simulink model "sgMdl_CAN_CounterAndCRC"  (R2024b)
settings: Solver=FixedStepAuto  StartTime=0.0  StopTime=inf  RelTol=1e-3  EnableMultiTasking=on
undefined symbols (not defined in the file): CAN, Down, FD, Pull
libraries: CAN_message_utilities x14, canfdmsglib x10, speedgoatlib_IO602_4 x9, simulink x4
Description:
  | CAN - Counter and CRC Message Protection
settings Model: ModifiedByFormat=Speedgoat  SimulationMode=external  ExtModeEnableFloating=off  ExtModeTrigDuration=100000  Creator=Speedgoat  LastModifiedBy=Speedgoat
settings SolverCC: ConcurrentTasks=on  AlgebraicLoopSolver=TrustRegion  PositivePriorityOrder=on  AutoInsertRateTranBlk=on  InsertRTBMode=Never (minimum delay)
settings DataIOCC: SaveFormat=StructureWithTime
settings OptimizationCC: BlockReduction=off  OptimizeBlockIOStorage=off  BufferReuse=off  GlobalBufferReuse=off  ExpressionFolding=off  LocalBlockOutputs=off  OptimizeDataStoreBuffers=off  BusAssignmentInplaceUpdate=off
settings DebuggingCC: InheritedTsInSrcMsg=none  TasksWithSamePriorityMsg=none  ParameterPrecisionLossMsg=none  UnconnectedInputMsg=warning  UnconnectedOutputMsg=warning  UnconnectedLineMsg=warning
settings HardwareCC: ProdBitPerLong=64  ProdLongLongMode=on  ProdHWDeviceType=Intel->x86-64 (Linux 64)
settings ModelReferenceCC: EnableRefExpFcnMdlSchedulingChecks=on
settings SFSimCC: CustomCodeUndefinedFunction=UseInterfaceOnly
settings RTWCC: Description=Speedgoat Real-Time Target Machine  SystemTargetFile=speedgoat.tlc  TemplateMakefile=slrealtime_default_tmf  Toolchain=Simulink Real-Time Toolchain  BuildConfiguration=Faster Runs  TargetLang=C++  GPUComputeCapability=3.5  DLArmComputeVersion=19.05
settings SimulinkRealTimeTargetCC: SubcomponentCodeInterfacePackaging=Reusable function  InstructionSetFMA=off  LogToMDFFile=off  SLRTFileLogMaxRuns=10  UseGCCFastMath=on
settings ConfigComp: CovBoundaryAbsTol=1.0e-5

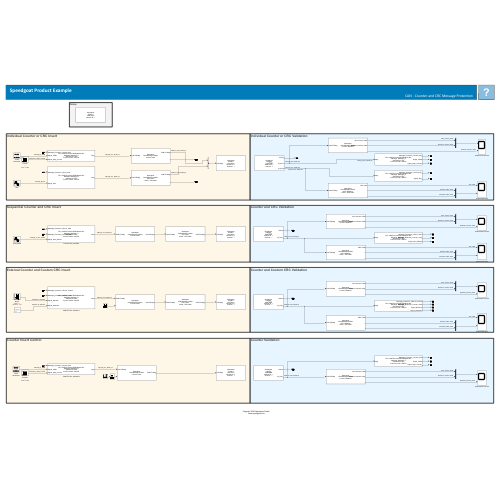
[thumbnail: Simulink's stored preview of the top-level diagram]
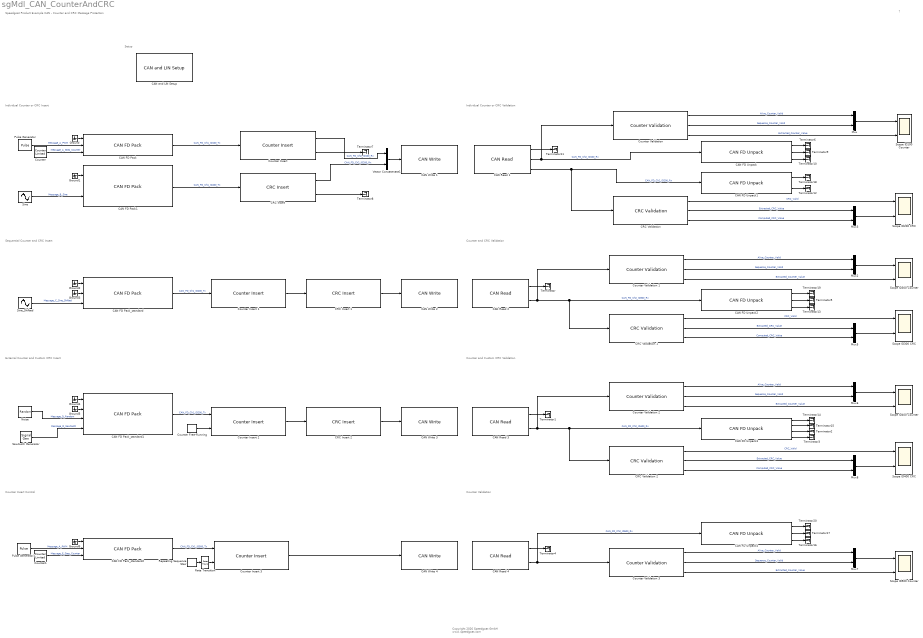
== system sgMdl_CAN_CounterAndCRC ==
  note: Individual Counter or CRC Insert
  note: Setup
  note: External Counter and Custom CRC Insert
  note: Counter Validation
  note: Individual Counter or CRC Validation
  note: Counter Insert Control
  note: Counter and CRC Validation
  note: Counter and Custom CRC Validation
  note: Sequential Counter and CRC Insert
  note: Speedgoat Product Example
      | CAN - Counter and CRC Message Protection
  note: ?
  note: Copyright 2026 Speedgoat GmbH
      |  www.speedgoat.com
  CAN FD Pack : canfdmsglib/CAN FD Pack  CANdbFile=CANFDCounterCRCDatabase.dbc  MsgList=Message_A  MsgName=Message_A  ProtocolMode=CAN FD  MsgIDType=Standard (11-bit identifier)  MsgIdentifier=100  CANIDInput=off  MsgLength=20  Remote=off  BRSSwitch=on  ApplyMinMax=off  SignalInfo={'Message_Protection_Counter_8bit','128','8','LE','unsigned','Standard','0','1','0','-Inf','Inf';'Signal_PWM','0','64','LE','double','Standard','0','1','0','-1.7e+308','1.7e+308';'Signal_Step_Counter','64','64','LE','double','Standard','0','1','0','-1.7e+308','1.7e+308'}
      settings: DataFormat=CANdb specified signals
  CAN FD Pack1 : canfdmsglib/CAN FD Pack  CANdbFile=CANFDCounterCRCDatabase.dbc  MsgList=Message_B  MsgName=Message_B  ProtocolMode=CAN FD  MsgIDType=Standard (11-bit identifier)  MsgIdentifier=200  CANIDInput=off  MsgLength=12  Remote=off  BRSSwitch=on  ApplyMinMax=off  SignalInfo={'Message_Protection_CRC8_0x2F','64','8','LE','unsigned','Standard','0','1','0','-Inf','Inf';'Signal_Sine','0','64','LE','double','Standard','0','1','0','-1.7e+308','1.7e+308'}
      settings: DataFormat=CANdb specified signals
  CAN FD Pack_standard : canfdmsglib/CAN FD Pack  CANdbFile=CANFDCounterCRCDatabase.dbc  MsgList=Message_C  MsgName=Message_C  ProtocolMode=CAN FD  MsgIDType=Standard (11-bit identifier)  MsgIdentifier=300  CANIDInput=off  MsgLength=12  Remote=off  BRSSwitch=on  ApplyMinMax=off  SignalInfo={'Message_Protection_CRC16_ARC','76','16','LE','unsigned','Standard','0','1','0','-Inf','Inf';'Message_Protection_Counter_12bit','64','12','LE','unsigned','Standard','0','1','0','-Inf','Inf';'Signal_Sine_Shifted','0','64','LE','double','Standard','0','1','0','-1.7e+308','1.7e+308'}
      settings: DataFormat=CANdb specified signals
  CAN FD Pack_standard1 : canfdmsglib/CAN FD Pack  CANdbFile=CANFDCounterCRCDatabase.dbc  MsgList=Message_D  MsgName=Message_D  ProtocolMode=CAN FD  MsgIDType=Standard (11-bit identifier)  MsgIdentifier=400  CANIDInput=off  MsgLength=7  Remote=off  BRSSwitch=on  ApplyMinMax=off  SignalInfo={'Message_Protection_CRC12_Custom','36','12','LE','unsigned','Standard','0','1','0','-Inf','Inf';'Message_Protection_Counter_16bit','12','16','LE','unsigned','Standard','0','1','0','-Inf','Inf';'Signal_Random','0','12','LE','unsigned','Standard','0','1','0','0','65535';'Signal_Sawtooth','28','6','LE','signed','Standard','0','1','0','-128','127'}
      settings: DataFormat=CANdb specified signals
  CAN FD Pack_standard2 : canfdmsglib/CAN FD Pack  CANdbFile=CANFDCounterCRCDatabase.dbc  MsgList=Message_E  MsgName=Message_E  ProtocolMode=CAN FD  MsgIDType=Standard (11-bit identifier)  MsgIdentifier=500  CANIDInput=off  MsgLength=20  Remote=off  BRSSwitch=on  ApplyMinMax=off  SignalInfo={'Message_Protection_Counter_8bit','128','8','LE','unsigned','Standard','0','1','0','-Inf','Inf';'Signal_PWM','0','64','LE','double','Standard','0','1','0','-1.7e+308','1.7e+308';'Signal_Step_Counter','64','64','LE','double','Standard','0','1','0','-1.7e+308','1.7e+308'}
      settings: DataFormat=CANdb specified signals
  CAN FD Unpack : canfdmsglib/CAN FD Unpack  CANdbFile=CANFDCounterCRCDatabase.dbc  MsgList=Message_A  MsgName=Message_A  ProtocolMode=CAN FD  MsgIDType=Standard (11-bit identifier)  MsgIdentifier=100  MsgLength=20  SignalInfo={'Message_Protection_Counter_8bit','128','8','LE','unsigned','Standard','0','1','0','-Inf','Inf';'Signal_PWM','0','64','LE','double','Standard','0','1','0','-1.7e+308','1.7e+308';'Signal_Step_Counter','64','64','LE','double','Standard','0','1','0','-1.7e+308','1.7e+308'}  IDPort=off  TimestampPort=off  ErrorPort=off  RemotePort=off  LengthPort=off  StatusPort=off  BRSPort=off  ESIPort=off  DLCPort=off  ApplyMinMax=off
      settings: DataFormat=CANdb specified signals
  CAN FD Unpack1 : canfdmsglib/CAN FD Unpack  CANdbFile=CANFDCounterCRCDatabase.dbc  MsgList=Message_B  MsgName=Message_B  ProtocolMode=CAN FD  MsgIDType=Standard (11-bit identifier)  MsgIdentifier=200  MsgLength=12  SignalInfo={'Message_Protection_CRC8_0x2F','64','8','LE','unsigned','Standard','0','1','0','-Inf','Inf';'Signal_Sine','0','64','LE','double','Standard','0','1','0','-1.7e+308','1.7e+308'}  IDPort=off  TimestampPort=off  ErrorPort=off  RemotePort=off  LengthPort=off  StatusPort=off  BRSPort=off  ESIPort=off  DLCPort=off  ApplyMinMax=off
      settings: DataFormat=CANdb specified signals
  CAN FD Unpack2 : canfdmsglib/CAN FD Unpack  CANdbFile=CANFDCounterCRCDatabase.dbc  MsgList=Message_C  MsgName=Message_C  ProtocolMode=CAN FD  MsgIDType=Standard (11-bit identifier)  MsgIdentifier=300  MsgLength=12  SignalInfo={'Message_Protection_CRC16_ARC','76','16','LE','unsigned','Standard','0','1','0','-Inf','Inf';'Message_Protection_Counter_12bit','64','12','LE','unsigned','Standard','0','1','0','-Inf','Inf';'Signal_Sine_Shifted','0','64','LE','double','Standard','0','1','0','-1.7e+308','1.7e+308'}  IDPort=off  TimestampPort=off  ErrorPort=off  RemotePort=off  LengthPort=off  StatusPort=off  BRSPort=off  ESIPort=off  DLCPort=off  ApplyMinMax=off
      settings: DataFormat=CANdb specified signals
  CAN FD Unpack3 : canfdmsglib/CAN FD Unpack  CANdbFile=CANFDCounterCRCDatabase.dbc  MsgList=Message_D  MsgName=Message_D  ProtocolMode=CAN FD  MsgIDType=Standard (11-bit identifier)  MsgIdentifier=400  MsgLength=7  SignalInfo={'Message_Protection_CRC12_Custom','36','12','LE','unsigned','Standard','0','1','0','-Inf','Inf';'Message_Protection_Counter_16bit','12','16','LE','unsigned','Standard','0','1','0','-Inf','Inf';'Signal_Random','0','12','LE','unsigned','Standard','0','1','0','0','65535';'Signal_Sawtooth','28','6','LE','signed','Standard','0','1','0','-128','127'}  IDPort=off  TimestampPort=off  ErrorPort=off  RemotePort=off  LengthPort=off  StatusPort=off  BRSPort=off  ESIPort=off  DLCPort=off  ApplyMinMax=off
      settings: DataFormat=CANdb specified signals
  CAN FD Unpack4 : canfdmsglib/CAN FD Unpack  CANdbFile=CANFDCounterCRCDatabase.dbc  MsgList=Message_E  MsgName=Message_E  ProtocolMode=CAN FD  MsgIDType=Standard (11-bit identifier)  MsgIdentifier=500  MsgLength=20  SignalInfo={'Message_Protection_Counter_8bit','128','8','LE','unsigned','Standard','0','1','0','-Inf','Inf';'Signal_PWM','0','64','LE','double','Standard','0','1','0','-1.7e+308','1.7e+308';'Signal_Step_Counter','64','64','LE','double','Standard','0','1','0','-1.7e+308','1.7e+308'}  IDPort=off  TimestampPort=off  ErrorPort=off  RemotePort=off  LengthPort=off  StatusPort=off  BRSPort=off  ESIPort=off  DLCPort=off  ApplyMinMax=off
      settings: DataFormat=CANdb specified signals
  CAN Read 1 : speedgoatlib_IO602_4/CAN Read   moduleType=IO603  id=1  channel=2  messageType=CAN-FD  useBusOut=on  HasMulRead=Specify by IDs  MsgIDlist=[100,200]  isEFF=off  LabelInHex=off  enableInput=off  initValues=[603 1 -1 1 2 0 1 2 0 2 100 200]  ts=-1
      settings: LibrarySourceBlock=speedgoatlib_IO602_IO691/CAN/CAN Read  SourceProductName=IO602-4
  CAN Read 2 : speedgoatlib_IO602_4/CAN Read   moduleType=IO603  id=1  channel=2  messageType=CAN-FD  useBusOut=on  HasMulRead=Specify by IDs  MsgIDlist=300  isEFF=off  LabelInHex=off  enableInput=off  initValues=[603 1 -1 1 2 0 1 2 0 1 300]  ts=-1
      settings: LibrarySourceBlock=speedgoatlib_IO602_IO691/CAN/CAN Read  SourceProductName=IO602-4
  CAN Read 3 : speedgoatlib_IO602_4/CAN Read   moduleType=IO603  id=1  channel=2  messageType=CAN-FD  useBusOut=on  HasMulRead=Specify by IDs  MsgIDlist=400  isEFF=off  LabelInHex=off  enableInput=off  initValues=[603 1 -1 1 2 0 1 2 0 1 400]  ts=-1
      settings: LibrarySourceBlock=speedgoatlib_IO602_IO691/CAN/CAN Read  SourceProductName=IO602-4
  CAN Read 4 : speedgoatlib_IO602_4/CAN Read   moduleType=IO603  id=1  channel=2  messageType=CAN-FD  useBusOut=on  HasMulRead=Specify by IDs  MsgIDlist=[500]  isEFF=off  LabelInHex=off  enableInput=off  initValues=[603 1 -1 1 2 0 1 2 0 1 500]  ts=-1
      settings: LibrarySourceBlock=speedgoatlib_IO602_IO691/CAN/CAN Read  SourceProductName=IO602-4
  CAN Write 1 : speedgoatlib_IO602_4/CAN Write   moduleType=IO603  id=1  channel=1  messageType=CAN-FD  useBusIn=on  numOfMsg=2  enableInput=off  enableStatusPort=off  ts=-1  initValues=[603 1 -1 0 2 0 2 0 1]
      settings: LibrarySourceBlock=speedgoatlib_IO602_IO691/CAN/CAN Write  SourceProductName=IO602-4
  CAN Write 2 : speedgoatlib_IO602_4/CAN Write   moduleType=IO603  id=1  channel=1  messageType=CAN-FD  useBusIn=on  numOfMsg=1  enableInput=off  enableStatusPort=off  ts=-1  initValues=[603 1 -1 0 2 0 1 0 1]
      settings: LibrarySourceBlock=speedgoatlib_IO602_IO691/CAN/CAN Write  SourceProductName=IO602-4
  CAN Write 3 : speedgoatlib_IO602_4/CAN Write   moduleType=IO603  id=1  channel=1  messageType=CAN-FD  useBusIn=on  numOfMsg=1  enableInput=off  enableStatusPort=off  ts=-1  initValues=[603 1 -1 0 2 0 1 0 1]
      settings: LibrarySourceBlock=speedgoatlib_IO602_IO691/CAN/CAN Write  SourceProductName=IO602-4
  CAN Write 4 : speedgoatlib_IO602_4/CAN Write   moduleType=IO603  id=1  channel=1  messageType=CAN-FD  useBusIn=on  numOfMsg=1  enableInput=off  enableStatusPort=off  ts=-1  initValues=[603 1 -1 0 2 0 1 0 1]
      settings: LibrarySourceBlock=speedgoatlib_IO602_IO691/CAN/CAN Write  SourceProductName=IO602-4
  "CAN and LIN Setup " : speedgoatlib_IO602_4/CAN and LIN Setup   moduleInitValues="[603    1    1   -1   -1]"  id=1  moduleType=IO603  pciSlot=-1  canChn1=CAN-FD  canChn2=CAN-FD  canChn3=Disabled  canChn4=Disabled  linChn1=Disabled  linChn2=Disabled  canInitStructArray=[]  canTermStructArray=[]  gpioChnx=Disabled  canChn1InitValues="[3   0   2   8  31   8  19   2   2   5   2   0]"  arbBdrChn1=1.0 MBaud  clockDividerChn1=Enable  arbManBdrChn1=[2,8,31,8]  fdBdrChn1=5.0 MBaud  fdManBdrChn1=[2,2,5,2]  termResistor1=off  canChn2InitValues="[3   0   2   8  31   8  19   2   2   5   2   0]"  arbBdrChn2=1.0 MBaud  clockDividerChn2=Enable  arbManBdrChn2=[2,8,31,8]  fdBdrChn2=5.0 MBaud  fdManBdrChn2=[2,2,5,2]  termResistor2=off  canChn3InitValues="[1   0   2   8  31   8  19   2   2   5   2   0]"  arbBdrChn3=1.0 MBaud  clockDividerChn3=Enable  arbManBdrChn3=[2,8,31,8]  fdBdrChn3=5.0 MBaud  fdManBdrChn3=[2,2,5,2]  termResistor3=off  canChn4InitValues="[1   0   2   8  31   8  19   2   2   5   2   0]"  arbBdrChn4=1.0 MBaud  clockDividerChn4=Enable  arbManBdrChn4=[2,8,31,8]  fdBdrChn4=5.0 MBaud  fdManBdrChn4=[2,2,5,2]  termResistor4=off  linChn1InitValues="[0  9600]"  linBtrChn1=9600  linChn2InitValues="[0  9600]"  linBtrChn2=9600  doInitTermStruct="[0  5  0  0  0]"  parDoChannels=[1 2]  parDoVoltage=5  parDoInitValues=0  parDoReset=1  parNumOfDoS=0  parDiChannels=[3 4]  parDiVoltage=5  parDiPull=Pull-Down
      settings: LibrarySourceBlock=speedgoatlib_IO602_IO691/CAN and LIN Setup  SourceProductName=IO602-4
  "CRC Insert " : CAN_message_utilities/CRC Insert   parEnableCrcPort=off  parCrcFromInput=off  parCrcOutput=on  parCrcType=CRC8 - 0x2F  parCrcBitLocation=64  parCustomCrcBitWidth=7  parCustomCrcFile=''  parCustomCrcFunction=''  parProtocol=CAN-FD  ts=-1  initValues=[0 2 47 255 255 0 0 64 1 7 2 -1]  lutParam=[0;47;94;113;188;147;226;205;87;120;9;38;235;196;181;154;174;129;240;223;18;61;76;99;249;214;167;136;69;106;27;52;115;92;45;2;207;224;145;190;36;11;122;85;152;183;198;233;221;242;131;172;97;78;63;16;138;165;212;251;54;25;104;71;230;201;184;151;90;117;4;43;177;158;239;192;13;34;83;124;72;103;22;57;244;219;170;133;31;48;65;110;163;140;253;210;149;186;203;228;41;6;119;88;194;237;156;179;126;81;32;15;59;20;101;74;135;168;217;246;108;67;50;29;208;255;142;161;227;204;189;146;95;112;1;46;180;155;234;197;8;39;86;121;77;98;19;60;241;222;175;128;26;53;68;107;166;137;248;215;144;191;206;225;44;3;114;93;199;232;153;182;123;84;37;10;62;17;96;79;130;173;220;243;105;70;55;24;213;250;139;164;5;42;91;116;185;150;231;200;82;125;12;35;238;193;176;159;171;132;245;218;23;56;73;102;252;211;162;141;64;111;30;49;118;89;40;7;202;229;148;187;33;14;127;80;157;178;195;236;216;247;134;169;100;75;58;21;143;160;209;254;51;28;109;66]
  CRC Insert 1 : CAN_message_utilities/CRC Insert   parEnableCrcPort=off  parCrcFromInput=off  parCrcOutput=off  parCrcType=CRC16 ARC  parCrcBitLocation=76  parCustomCrcBitWidth=7  parCustomCrcFile='test'  parCustomCrcFunction=''  parProtocol=CAN-FD  ts=-1  initValues=[0 5 32773 0 0 1 1 76 0 7 2 -1]  lutParam=[0;32773;32783;10;32795;30;20;32785;32819;54;60;32825;40;32813;32807;34;32867;102;108;32873;120;32893;32887;114;80;32853;32863;90;32843;78;68;32833;32963;198;204;32969;216;32989;32983;210;240;33013;33023;250;33003;238;228;32993;160;32933;32943;170;32955;190;180;32945;32915;150;156;32921;136;32909;32903;130;33155;390;396;33161;408;33181;33175;402;432;33205;33215;442;33195;430;420;33185;480;33253;33263;490;33275;510;500;33265;33235;470;476;33241;456;33229;33223;450;320;33093;33103;330;33115;350;340;33105;33139;374;380;33145;360;33133;33127;354;33059;294;300;33065;312;33085;33079;306;272;33045;33055;282;33035;270;260;33025;33539;774;780;33545;792;33565;33559;786;816;33589;33599;826;33579;814;804;33569;864;33637;33647;874;33659;894;884;33649;33619;854;860;33625;840;33613;33607;834;960;33733;33743;970;33755;990;980;33745;33779;1014;1020;33785;1000;33773;33767;994;33699;934;940;33705;952;33725;33719;946;912;33685;33695;922;33675;910;900;33665;640;33413;33423;650;33435;670;660;33425;33459;694;700;33465;680;33453;33447;674;33507;742;748;33513;760;33533;33527;754;720;33493;33503;730;33483;718;708;33473;33347;582;588;33353;600;33373;33367;594;624;33397;33407;634;33387;622;612;33377;544;33317;33327;554;33339;574;564;33329;33299;534;540;33305;520;33293;33287;514]
  CRC Insert 2 : CAN_message_utilities/CRC Insert   parEnableCrcPort=off  parCrcFromInput=on  parCrcOutput=off  parCrcType=Custom  parCrcBitLocation=36  parCustomCrcBitWidth=12  parCustomCrcFile='custom_crc.cpp'  parCustomCrcFunction='ComputeCustomCrc'  parProtocol=CAN-FD  ts=-1  initValues=[0 8 0 0 0 0 0 36 0 12 2 -1]  lutParam=[0;29;58;39;116;105;78;83;232;245;210;207;156;129;166;187;205;208;247;234;185;164;131;158;37;56;31;2;81;76;107;118;135;154;189;160;243;238;201;212;111;114;85;72;27;6;33;60;74;87;112;109;62;35;4;25;162;191;152;133;214;203;236;241;19;14;41;52;103;122;93;64;251;230;193;220;143;146;181;168;222;195;228;249;170;183;144;141;54;43;12;17;66;95;120;101;148;137;174;179;224;253;218;199;124;97;70;91;8;21;50;47;89;68;99;126;45;48;23;10;177;172;139;150;197;216;255;226;38;59;28;1;82;79;104;117;206;211;244;233;186;167;128;157;235;246;209;204;159;130;165;184;3;30;57;36;119;106;77;80;161;188;155;134;213;200;239;242;73;84;115;110;61;32;7;26;108;113;86;75;24;5;34;63;132;153;190;163;240;237;202;215;53;40;15;18;65;92;123;102;221;192;231;250;169;180;147;142;248;229;194;223;140;145;182;171;16;13;42;55;100;121;94;67;178;175;136;149;198;219;252;225;90;71;96;125;46;51;20;9;127;98;69;88;11;22;49;44;151;138;173;176;227;254;217;196]
  "CRC Validation " : CAN_message_utilities/CRC Validation   parEnableCrcPort=off  parCrcFromInput=off  parComputedCrcOutput=on  parExtractedCrcOutput=on  parCrcValidOutput=on  parCrcType=CRC8 - 0x2F  parCrcBitLocation=64  parCustomCrcBitWidth=8  parCustomCrcFile=''  parCustomCrcFunction=''  parProtocol=CAN-FD  ts=-1  initValues=[0 2 47 255 255 0 0 64 1 1 1 8 2 -1]  lutParam=[0;47;94;113;188;147;226;205;87;120;9;38;235;196;181;154;174;129;240;223;18;61;76;99;249;214;167;136;69;106;27;52;115;92;45;2;207;224;145;190;36;11;122;85;152;183;198;233;221;242;131;172;97;78;63;16;138;165;212;251;54;25;104;71;230;201;184;151;90;117;4;43;177;158;239;192;13;34;83;124;72;103;22;57;244;219;170;133;31;48;65;110;163;140;253;210;149;186;203;228;41;6;119;88;194;237;156;179;126;81;32;15;59;20;101;74;135;168;217;246;108;67;50;29;208;255;142;161;227;204;189;146;95;112;1;46;180;155;234;197;8;39;86;121;77;98;19;60;241;222;175;128;26;53;68;107;166;137;248;215;144;191;206;225;44;3;114;93;199;232;153;182;123;84;37;10;62;17;96;79;130;173;220;243;105;70;55;24;213;250;139;164;5;42;91;116;185;150;231;200;82;125;12;35;238;193;176;159;171;132;245;218;23;56;73;102;252;211;162;141;64;111;30;49;118;89;40;7;202;229;148;187;33;14;127;80;157;178;195;236;216;247;134;169;100;75;58;21;143;160;209;254;51;28;109;66]
  CRC Validation 1 : CAN_message_utilities/CRC Validation   parEnableCrcPort=off  parCrcFromInput=off  parComputedCrcOutput=on  parExtractedCrcOutput=on  parCrcValidOutput=on  parCrcType=CRC16 ARC  parCrcBitLocation=76  parCustomCrcBitWidth=8  parCustomCrcFile=''  parCustomCrcFunction=''  parProtocol=CAN-FD  ts=-1  initValues=[0 5 32773 0 0 1 1 76 1 1 1 8 2 -1]  lutParam=[0;32773;32783;10;32795;30;20;32785;32819;54;60;32825;40;32813;32807;34;32867;102;108;32873;120;32893;32887;114;80;32853;32863;90;32843;78;68;32833;32963;198;204;32969;216;32989;32983;210;240;33013;33023;250;33003;238;228;32993;160;32933;32943;170;32955;190;180;32945;32915;150;156;32921;136;32909;32903;130;33155;390;396;33161;408;33181;33175;402;432;33205;33215;442;33195;430;420;33185;480;33253;33263;490;33275;510;500;33265;33235;470;476;33241;456;33229;33223;450;320;33093;33103;330;33115;350;340;33105;33139;374;380;33145;360;33133;33127;354;33059;294;300;33065;312;33085;33079;306;272;33045;33055;282;33035;270;260;33025;33539;774;780;33545;792;33565;33559;786;816;33589;33599;826;33579;814;804;33569;864;33637;33647;874;33659;894;884;33649;33619;854;860;33625;840;33613;33607;834;960;33733;33743;970;33755;990;980;33745;33779;1014;1020;33785;1000;33773;33767;994;33699;934;940;33705;952;33725;33719;946;912;33685;33695;922;33675;910;900;33665;640;33413;33423;650;33435;670;660;33425;33459;694;700;33465;680;33453;33447;674;33507;742;748;33513;760;33533;33527;754;720;33493;33503;730;33483;718;708;33473;33347;582;588;33353;600;33373;33367;594;624;33397;33407;634;33387;622;612;33377;544;33317;33327;554;33339;574;564;33329;33299;534;540;33305;520;33293;33287;514]
  CRC Validation 2 : CAN_message_utilities/CRC Validation   parEnableCrcPort=off  parCrcFromInput=off  parComputedCrcOutput=on  parExtractedCrcOutput=on  parCrcValidOutput=on  parCrcType=Custom  parCrcBitLocation=36  parCustomCrcBitWidth=12  parCustomCrcFile='custom_crc.cpp'  parCustomCrcFunction='ComputeCustomCrc'  parProtocol=CAN-FD  ts=-1  initValues=[0 8 0 0 0 0 0 36 1 1 1 12 2 -1]  lutParam=[0;47;94;113;188;147;226;205;87;120;9;38;235;196;181;154;174;129;240;223;18;61;76;99;249;214;167;136;69;106;27;52;115;92;45;2;207;224;145;190;36;11;122;85;152;183;198;233;221;242;131;172;97;78;63;16;138;165;212;251;54;25;104;71;230;201;184;151;90;117;4;43;177;158;239;192;13;34;83;124;72;103;22;57;244;219;170;133;31;48;65;110;163;140;253;210;149;186;203;228;41;6;119;88;194;237;156;179;126;81;32;15;59;20;101;74;135;168;217;246;108;67;50;29;208;255;142;161;227;204;189;146;95;112;1;46;180;155;234;197;8;39;86;121;77;98;19;60;241;222;175;128;26;53;68;107;166;137;248;215;144;191;206;225;44;3;114;93;199;232;153;182;123;84;37;10;62;17;96;79;130;173;220;243;105;70;55;24;213;250;139;164;5;42;91;116;185;150;231;200;82;125;12;35;238;193;176;159;171;132;245;218;23;56;73;102;252;211;162;141;64;111;30;49;118;89;40;7;202;229;148;187;33;14;127;80;157;178;195;236;216;247;134;169;100;75;58;21;143;160;209;254;51;28;109;66]
  Counter : simulink/Sources/Counter Limited  uplimit=64  tsamp=10e-3
      settings: AttributesFormatString=|
      | ---
      | Limit: %<uplimit> bits
  Counter Free-Running : simulink/Sources/Counter Free-Running  NumBits=16  tsamp=10e-3
  "Counter Insert " : CAN_message_utilities/Counter Insert   parEnablePort=off  parCounterControlPort=off  parCounterFromInput=off  parCounterOutport=on  parCounterStart=1  parCounterStop=15  parCounterStep=1  parCounterBitLocation=128  parCounterLength=8  parProtocol=CAN-FD  ts=-1  initValues=[0 0 0 1 15 1 128 8 1 2 -1]
  Counter Insert 1 : CAN_message_utilities/Counter Insert   parEnablePort=off  parCounterControlPort=off  parCounterFromInput=off  parCounterOutport=off  parCounterStart=1  parCounterStop=4000  parCounterStep=3  parCounterBitLocation=64  parCounterLength=12  parProtocol=CAN-FD  ts=-1  initValues=[0 0 0 1 4000 3 64 12 0 2 -1]
  Counter Insert 2 : CAN_message_utilities/Counter Insert   parEnablePort=off  parCounterControlPort=off  parCounterFromInput=on  parCounterOutport=off  parCounterStart=1  parCounterStop=15  parCounterStep=1  parCounterBitLocation=12  parCounterLength=16  parProtocol=CAN-FD  ts=-1  initValues=[0 0 1 1 15 1 12 16 0 2 -1]
  Counter Insert 3 : CAN_message_utilities/Counter Insert   parEnablePort=off  parCounterControlPort=on  parCounterFromInput=off  parCounterOutport=off  parCounterStart=1  parCounterStop=15  parCounterStep=1  parCounterBitLocation=128  parCounterLength=8  parProtocol=CAN-FD  ts=-1  initValues=[0 1 0 1 15 1 128 8 0 2 -1]
  "Counter Validation " : CAN_message_utilities/Counter Validation   parExtractedCounterOutput=on  parAliveCounterValidOutput=on  parSequenceCounterValidOutput=on  parMissedFramesOutput=off  parCounterStartValue=1  parCounterStopValue=15  parCounterStepValue=1  parCounterBitLocation=128  parCounterBitWidth=8  parProtocol=CAN-FD  ts=-1  initValues=[1 15 1 128 8 1 1 1 0 2 -1]  lutParam=[0;29;58;39;116;105;78;83;232;245;210;207;156;129;166;187;205;208;247;234;185;164;131;158;37;56;31;2;81;76;107;118;135;154;189;160;243;238;201;212;111;114;85;72;27;6;33;60;74;87;112;109;62;35;4;25;162;191;152;133;214;203;236;241;19;14;41;52;103;122;93;64;251;230;193;220;143;146;181;168;222;195;228;249;170;183;144;141;54;43;12;17;66;95;120;101;148;137;174;179;224;253;218;199;124;97;70;91;8;21;50;47;89;68;99;126;45;48;23;10;177;172;139;150;197;216;255;226;38;59;28;1;82;79;104;117;206;211;244;233;186;167;128;157;235;246;209;204;159;130;165;184;3;30;57;36;119;106;77;80;161;188;155;134;213;200;239;242;73;84;115;110;61;32;7;26;108;113;86;75;24;5;34;63;132;153;190;163;240;237;202;215;53;40;15;18;65;92;123;102;221;192;231;250;169;180;147;142;248;229;194;223;140;145;182;171;16;13;42;55;100;121;94;67;178;175;136;149;198;219;252;225;90;71;96;125;46;51;20;9;127;98;69;88;11;22;49;44;151;138;173;176;227;254;217;196]
  Counter Validation 1 : CAN_message_utilities/Counter Validation   parExtractedCounterOutput=on  parAliveCounterValidOutput=on  parSequenceCounterValidOutput=on  parMissedFramesOutput=off  parCounterStartValue=1  parCounterStopValue=4000  parCounterStepValue=3  parCounterBitLocation=64  parCounterBitWidth=12  parProtocol=CAN-FD  ts=-1  initValues=[1 4000 3 64 12 1 1 1 0 2 -1]  lutParam=[0;29;58;39;116;105;78;83;232;245;210;207;156;129;166;187;205;208;247;234;185;164;131;158;37;56;31;2;81;76;107;118;135;154;189;160;243;238;201;212;111;114;85;72;27;6;33;60;74;87;112;109;62;35;4;25;162;191;152;133;214;203;236;241;19;14;41;52;103;122;93;64;251;230;193;220;143;146;181;168;222;195;228;249;170;183;144;141;54;43;12;17;66;95;120;101;148;137;174;179;224;253;218;199;124;97;70;91;8;21;50;47;89;68;99;126;45;48;23;10;177;172;139;150;197;216;255;226;38;59;28;1;82;79;104;117;206;211;244;233;186;167;128;157;235;246;209;204;159;130;165;184;3;30;57;36;119;106;77;80;161;188;155;134;213;200;239;242;73;84;115;110;61;32;7;26;108;113;86;75;24;5;34;63;132;153;190;163;240;237;202;215;53;40;15;18;65;92;123;102;221;192;231;250;169;180;147;142;248;229;194;223;140;145;182;171;16;13;42;55;100;121;94;67;178;175;136;149;198;219;252;225;90;71;96;125;46;51;20;9;127;98;69;88;11;22;49;44;151;138;173;176;227;254;217;196]
  Counter Validation 2 : CAN_message_utilities/Counter Validation   parExtractedCounterOutput=on  parAliveCounterValidOutput=on  parSequenceCounterValidOutput=on  parMissedFramesOutput=off  parCounterStartValue=0  parCounterStopValue=65535  parCounterStepValue=1  parCounterBitLocation=12  parCounterBitWidth=16  parProtocol=CAN-FD  ts=-1  initValues=[0 65535 1 12 16 1 1 1 0 2 -1]  lutParam=[0;29;58;39;116;105;78;83;232;245;210;207;156;129;166;187;205;208;247;234;185;164;131;158;37;56;31;2;81;76;107;118;135;154;189;160;243;238;201;212;111;114;85;72;27;6;33;60;74;87;112;109;62;35;4;25;162;191;152;133;214;203;236;241;19;14;41;52;103;122;93;64;251;230;193;220;143;146;181;168;222;195;228;249;170;183;144;141;54;43;12;17;66;95;120;101;148;137;174;179;224;253;218;199;124;97;70;91;8;21;50;47;89;68;99;126;45;48;23;10;177;172;139;150;197;216;255;226;38;59;28;1;82;79;104;117;206;211;244;233;186;167;128;157;235;246;209;204;159;130;165;184;3;30;57;36;119;106;77;80;161;188;155;134;213;200;239;242;73;84;115;110;61;32;7;26;108;113;86;75;24;5;34;63;132;153;190;163;240;237;202;215;53;40;15;18;65;92;123;102;221;192;231;250;169;180;147;142;248;229;194;223;140;145;182;171;16;13;42;55;100;121;94;67;178;175;136;149;198;219;252;225;90;71;96;125;46;51;20;9;127;98;69;88;11;22;49;44;151;138;173;176;227;254;217;196]
  Counter Validation 3 : CAN_message_utilities/Counter Validation   parExtractedCounterOutput=on  parAliveCounterValidOutput=on  parSequenceCounterValidOutput=on  parMissedFramesOutput=off  parCounterStartValue=1  parCounterStopValue=15  parCounterStepValue=1  parCounterBitLocation=128  parCounterBitWidth=8  parProtocol=CAN-FD  ts=-1  initValues=[1 15 1 128 8 1 1 1 0 2 -1]  lutParam=[0;29;58;39;116;105;78;83;232;245;210;207;156;129;166;187;205;208;247;234;185;164;131;158;37;56;31;2;81;76;107;118;135;154;189;160;243;238;201;212;111;114;85;72;27;6;33;60;74;87;112;109;62;35;4;25;162;191;152;133;214;203;236;241;19;14;41;52;103;122;93;64;251;230;193;220;143;146;181;168;222;195;228;249;170;183;144;141;54;43;12;17;66;95;120;101;148;137;174;179;224;253;218;199;124;97;70;91;8;21;50;47;89;68;99;126;45;48;23;10;177;172;139;150;197;216;255;226;38;59;28;1;82;79;104;117;206;211;244;233;186;167;128;157;235;246;209;204;159;130;165;184;3;30;57;36;119;106;77;80;161;188;155;134;213;200;239;242;73;84;115;110;61;32;7;26;108;113;86;75;24;5;34;63;132;153;190;163;240;237;202;215;53;40;15;18;65;92;123;102;221;192;231;250;169;180;147;142;248;229;194;223;140;145;182;171;16;13;42;55;100;121;94;67;178;175;136;149;198;219;252;225;90;71;96;125;46;51;20;9;127;98;69;88;11;22;49;44;151;138;173;176;227;254;217;196]
  Counter1 : simulink/Sources/Counter Limited  uplimit=64  tsamp=10e-3
      settings: AttributesFormatString=|
      | ---
      | Limit: %<uplimit> bits
  Ground{,1..6} (7 alike) : Ground
  Mux{,2..3,5..8} (7 alike) : Mux  Inputs=2
  Noise : RandomNumber  Variance=100  SampleTime=10e-3
      settings: AttributesFormatString=|
      | Mean: %<Mean>
      | Variance: %<Variance>
  Pulse Generator : DiscretePulseGenerator  Period=50  PulseWidth=20  SampleTime=10e-3
  Pulse Generator1 : DiscretePulseGenerator  Period=50  PulseWidth=20  SampleTime=10e-3
  Rate Transition : RateTransition
  Repeating Sequence Stair : simulink/Sources/Repeating Sequence Stair  OutValues=[1 0 5 0xFFFF].'  tsamp=1  OutMin=[]  OutMax=[]  OutDataTypeStr=uint32  OutputDataTypeScalingMode=uint32  OutDataType=fixdt(0,8)  ConRadixGroup=Best Precision: Vector-wise  OutScaling=2^-12
  Sawtooth Generator : SignalGenerator  WaveForm=sawtooth  Amplitude=63  Frequency=5
  Scope ID100 Counter : Scope  NumInputPorts=2
  Scope ID200 CRC : Scope  NumInputPorts=2
  Scope ID300 CRC : Scope  NumInputPorts=2
  Scope ID300 Counter : Scope  NumInputPorts=2
  Scope ID400 CRC : Scope  NumInputPorts=2
  Scope ID400 Counter : Scope  NumInputPorts=2
  Scope ID500 Counter : Scope  NumInputPorts=2
  Sine : Sin  Amplitude=255  Frequency=2*pi  SampleTime=10e-3
  Sine_Shifted : Sin  Amplitude=255  Bias=pi  Frequency=2*pi  SampleTime=10e-3
  Terminator{,1..20} (21 alike) : Terminator
  Vector Concatenate1 : Concatenate
  wires:
  "Counter Validation "/3 -> Scope ID100 Counter/2  "Extracted_Counter_Value"
  CRC Validation 1/2 -> Mux5/1  "Extracted_CRC_Value"
  "CRC Validation "/1 -> Scope ID200 CRC/1  "CRC_Valid"
  CAN FD Unpack2/3 -> Terminator13/1
  CAN Read 3/1 -> Terminator1/1
  CAN Read 2/2 -> CRC Validation 1/1, CAN FD Unpack2/1, Counter Validation 1/1  "CAN_FD_Ch2_ID300_Rx"
  CAN FD Unpack/2 -> Terminator9/1
  CAN Read 1/2 -> "Counter Validation "/1, CAN FD Unpack/1  "CAN_FD_Ch2_ID100_Rx"
  CAN Read 1/1 -> Terminator11/1
  CAN FD Pack_standard1/1 -> Counter Insert 2/1  "CAN_FD_Ch1_ID200_Tx"
  CAN FD Unpack/1 -> Terminator6/1
  Pulse Generator/1 -> CAN FD Pack/2  "Message_A_PWM"
  CAN FD Pack1/1 -> "CRC Insert "/1  "CAN_FD_Ch1_ID400_Tx"
  CRC Validation 1/1 -> Scope ID300 CRC/1  "CRC_Valid"
  Counter/1 -> CAN FD Pack/3  "Message_A_Step_Counter"
  "Counter Insert "/2 -> Terminator7/1
  "CRC Validation "/2 -> Mux3/1  "Extracted_CRC_Value"
  Counter Validation 2/2 -> Mux6/2  "Sequence_Counter_Valid"
  Counter Validation 1/1 -> Mux2/1  "Alive_Counter_Valid"
  Noise/1 -> CAN FD Pack_standard1/3  "Message_D_Random"
  Mux6/1 -> Scope ID400 Counter/1
  CAN Read 2/1 -> Terminator/1
  Ground5/1 -> CAN FD Pack_standard1/2
  Ground2/1 -> CAN FD Pack_standard/1
  Counter Validation 2/1 -> Mux6/1  "Alive_Counter_Valid"
  Sine_Shifted/1 -> CAN FD Pack_standard/3  "Message_C_Sine_Shifted"
  CRC Validation 2/3 -> Mux8/2  "Computed_CRC_Value"
  CAN FD Unpack3/3 -> Terminator2/1
  Mux/1 -> Scope ID100 Counter/1
  Mux2/1 -> Scope ID300 Counter/1
  CAN FD Unpack3/1 -> Terminator14/1
  Ground1/1 -> CAN FD Pack1/1
  "CRC Validation "/3 -> Mux3/2  "Computed_CRC_Value"
  Sine/1 -> CAN FD Pack1/2  "Message_B_Sine"
  CAN FD Pack_standard/1 -> Counter Insert 1/1  "CAN_FD_Ch1_ID200_Tx"
  Ground3/1 -> CAN FD Pack_standard/2
  CAN FD Unpack3/2 -> Terminator15/1
  Counter Validation 1/3 -> Scope ID300 Counter/2  "Extracted_Counter_Value"
  CAN FD Pack_standard2/1 -> Counter Insert 3/1  "CAN_FD_Ch1_ID500_Tx"
  "Counter Validation "/2 -> Mux/2  "Sequence_Counter_Valid"
  Mux5/1 -> Scope ID300 CRC/2
  Repeating Sequence Stair/1 -> Rate Transition/1
  CAN FD Unpack3/4 -> Terminator3/1
  Mux8/1 -> Scope ID400 CRC/2
  CAN FD Unpack1/2 -> Terminator12/1
  "CRC Insert "/2 -> Terminator8/1
  Mux3/1 -> Scope ID200 CRC/2
  Counter Validation 2/3 -> Scope ID400 Counter/2  "Extracted_Counter_Value"
  Vector Concatenate1/1 -> CAN Write 1/1
  CAN Read 1/3 -> "CRC Validation "/1, CAN FD Unpack1/1  "CAN_FD_Ch2_ID200_Rx"
  CAN FD Unpack1/1 -> Terminator18/1
  CAN FD Pack/1 -> "Counter Insert "/1  "CAN_FD_Ch1_ID100_Tx"
  CRC Validation 2/1 -> Scope ID400 CRC/1  "CRC_Valid"
  Sawtooth Generator/1 -> CAN FD Pack_standard1/4  "Message_D_Sawtooth"
  CAN FD Unpack2/2 -> Terminator5/1
  CRC Validation 1/3 -> Mux5/2  "Computed_CRC_Value"
  Ground4/1 -> CAN FD Pack_standard1/1
  Counter Insert 1/1 -> CRC Insert 1/1
  CAN Read 3/2 -> CRC Validation 2/1, CAN FD Unpack3/1, Counter Validation 2/1  "CAN_FD_Ch2_ID400_Rx"
  CRC Validation 2/2 -> Mux8/1  "Extracted_CRC_Value"
  "Counter Validation "/1 -> Mux/1  "Alive_Counter_Valid"
  CAN FD Unpack/3 -> Terminator10/1
  Ground/1 -> CAN FD Pack/1
  Counter Validation 1/2 -> Mux2/2  "Sequence_Counter_Valid"
  Counter Validation 3/3 -> Scope ID500 Counter/2  "Extracted_Counter_Value"
  CAN FD Unpack4/2 -> Terminator17/1
  Counter Validation 3/2 -> Mux7/2  "Sequence_Counter_Valid"
  CAN FD Unpack4/3 -> Terminator16/1
  Mux7/1 -> Scope ID500 Counter/1
  CAN FD Unpack4/1 -> Terminator20/1
  Counter Validation 3/1 -> Mux7/1  "Alive_Counter_Valid"
  CAN Read 4/2 -> CAN FD Unpack4/1, Counter Validation 3/1  "CAN_FD_Ch2_ID500_Rx"
  CAN Read 4/1 -> Terminator4/1
  Pulse Generator1/1 -> CAN FD Pack_standard2/2  "Message_A_PWM"
  Counter1/1 -> CAN FD Pack_standard2/3  "Message_E_Step_Counter"
  Ground6/1 -> CAN FD Pack_standard2/1
  Counter Free-Running/1 -> Counter Insert 2/2
  Counter Insert 2/1 -> CRC Insert 2/1
  CAN FD Unpack2/1 -> Terminator19/1
  "Counter Insert "/1 -> Vector Concatenate1/1  "CAN_FD_Ch2_ID100_Rx"
  "CRC Insert "/1 -> Vector Concatenate1/2  "CAN_FD_Ch2_ID200_Rx"
  CRC Insert 1/1 -> CAN Write 2/1
  CRC Insert 2/1 -> CAN Write 3/1
  Counter Insert 3/1 -> CAN Write 4/1
  Rate Transition/1 -> Counter Insert 3/2
